simulink model "transientResponseRLCsquareWave"  (R2013a)
settings: Solver=ode45  StartTime=0.0  StopTime=0.0002  MaxStep=1e-4  RelTol=1e-5
libraries: powerlib x9
settings Model: Creator=dell pc  LastModifiedBy=hp

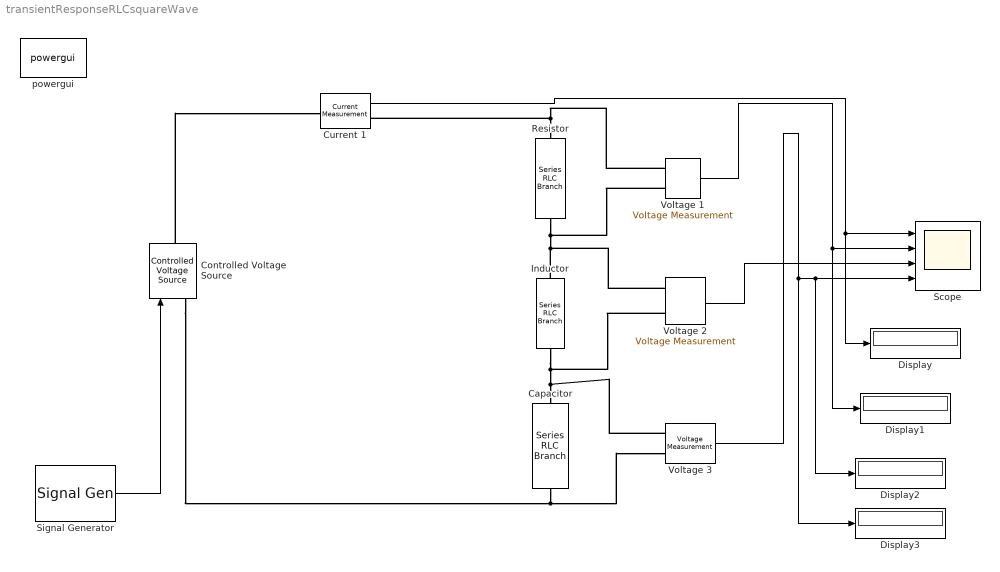
== system transientResponseRLCsquareWave ==
  Capacitor : powerlib/Elements/Series RLC Branch  LConnTagsString=__new0  RConnTagsString=__new0  BranchType=C  Resistance=1  Inductance=1e-3  SetiL0=off  InitialCurrent=0  Capacitance=0.05e-6  Setx0=off  InitialVoltage=0  Measurements=Branch voltage and current
  Controlled Voltage Source : powerlib/Electrical Sources/Controlled Voltage Source  Initialize=on  Source_Type=AC  Amplitude=0  Phase=0  Frequency=0.05  Measurements=None
  Current 1 : powerlib/Measurements/Current Measurement  PhasorSimulation=off  OutputType=Complex  PSBequivalent=0
  Display{,1..3} (4 alike) : Display
  Inductor : powerlib/Elements/Series RLC Branch  LConnTagsString=__new0  RConnTagsString=__new0  BranchType=L  Resistance=1  Inductance=1e-3  SetiL0=off  InitialCurrent=0  Capacitance=1e-6  Setx0=off  InitialVoltage=0  Measurements=None
  "Resistor " : powerlib/Elements/Series RLC Branch  LConnTagsString=__new0  RConnTagsString=__new0  BranchType=R  Resistance=20  Inductance=1e-3  SetiL0=off  InitialCurrent=0  Capacitance=1e-6  Setx0=off  InitialVoltage=0  Measurements=Branch voltage and current
  Scope : Scope  NumInputPorts=4
      settings: TimeRange=0.0001  YMin=-5~-5~-5~-5  YMax=5~5~5~5  SaveName=tt
  Signal Generator : SignalGenerator  WaveForm=square  Amplitude=20  Frequency=0.05
  Voltage 1 : powerlib/Measurements/Voltage Measurement  PhasorSimulation=off  OutputType=Complex  PSBequivalent=0
  Voltage 2 : powerlib/Measurements/Voltage Measurement  PhasorSimulation=off  OutputType=Complex  PSBequivalent=0
  Voltage 3 : powerlib/Measurements/Voltage Measurement  PhasorSimulation=off  OutputType=Complex  PSBequivalent=0
  powergui : powerlib/powergui  Priority=1  SimulationMode=Continuous  SolverType=Tustin  SampleTime=50e-6  frequency=60  SPID=off  DisableSnubberDevices=off  DisableRonSwitches=off  DisableVfSwitches=off  SwTol=0  Interpol=off  DisplayEquations=off  frequencyindice=0.05  Pbase=100e6  ErrMax=1e-4  Iterations=50  UnitsV=kV  UnitsW=MW  FunctionMessages=off  echomessages=off  HookPort=off  EnableUseOfTLC=off  x0status=blocks  RestoreLinks=warning  ResistiveCurrentMeasurement=off  Frange=[0:2:500]  Ylog=off  Xlog=on  ShowGrid=off  save=off  variable=ZData  ZoomFFT=off  StartTime=0.0  cycles=1  DisplayStyle=1  fundamental=60  FreqAxis=off  MaxFrequency=1000  frequencyindicesteady=1  RmsSteady=1  display=off  Ts=0  methode=off
  wires:
  Signal Generator/1 -> Controlled Voltage Source/1
  Voltage 3/1 -> Display3/1, Display2/1, Scope/4
  Voltage 1/1 -> Display1/1, Scope/2
  Current 1/1 -> Scope/1, Display/1
  Voltage 2/1 -> Scope/3
  connections:
  "Resistor "/RConn1 -- Inductor/LConn1 -- Voltage 2/LConn1 -- Voltage 1/LConn2
  Voltage 2/LConn2 -- Voltage 3/LConn1 -- Capacitor/LConn1 -- Inductor/RConn1
  Controlled Voltage Source/RConn1 -- Current 1/LConn1
  Controlled Voltage Source/LConn1 -- Voltage 3/LConn2 -- Capacitor/RConn1
  Voltage 1/LConn1 -- "Resistor "/LConn1 -- Current 1/RConn1
